simulink model "Parameter_Estimation"  (R2025a)
settings: Solver=FixedStepAuto  StartTime=0.0  StopTime=10  FixedStep=0.001  RelTol=1e-3
values from neighbouring files (symbols this model uses):
  C = 0.1    [parameter.m]
  K = 0.625    [parameter.m]
  m = 0.1    [parameter.m]
  x0 = 18    [parameter.m]
settings Model: Creator=tanawatp  LastModifiedBy=rajap
settings RTWCC: GPUComputeCapability=3.5

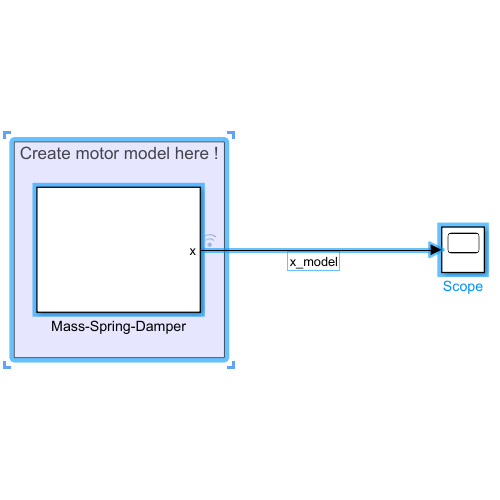
[thumbnail: Simulink's stored preview of the top-level diagram]
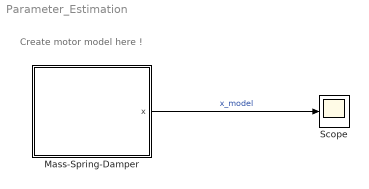
== system Parameter_Estimation ==
  note: Create motor model here !
  Mass-Spring-Damper : Subsystem
  Scope : Scope
      settings: ActiveDisplayYMinimum=-14.968704955703449  ActiveDisplayYMaximum=26.782665696383475
  wires:
  Mass-Spring-Damper/1(x) -> Scope/1  "x_model"

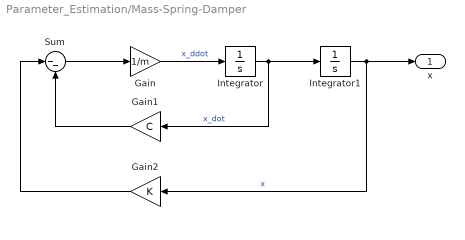
== system Parameter_Estimation/Mass-Spring-Damper ==
  Gain : Gain  Gain=1/m
  Gain1 : Gain  Gain=C
  Gain2 : Gain  Gain=K
  Integrator : Integrator
  Integrator1 : Integrator  InitialCondition=x0
  Sum : Sum  Inputs=|--
  x : Outport
  wires:
  Sum/1 -> Gain/1
  Gain/1 -> Integrator/1  "x_ddot"
  Integrator/1 -> Gain1/1, Integrator1/1  "x_dot"
  Gain1/1 -> Sum/2
  Integrator1/1 -> Gain2/1, x/1  "x"
  Gain2/1 -> Sum/1
